simulink model "sampleModel1440"  (R2023a)
settings: Solver=VariableStepAuto  StartTime=0.0  StopTime=10.0  RelTol=1e-3
libraries: hdlsllib x3
settings Model: Creator=user1  LastModifiedBy=user1

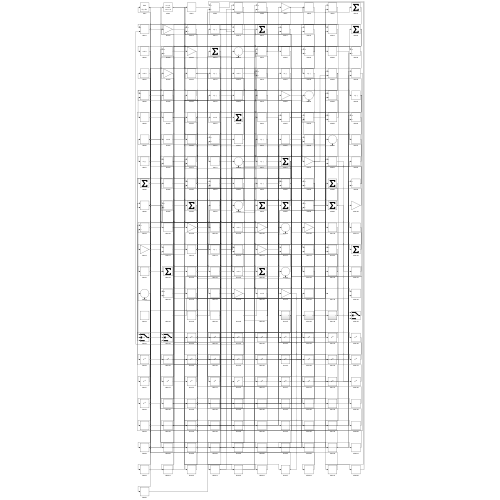
[thumbnail: Simulink's stored preview of the top-level diagram]
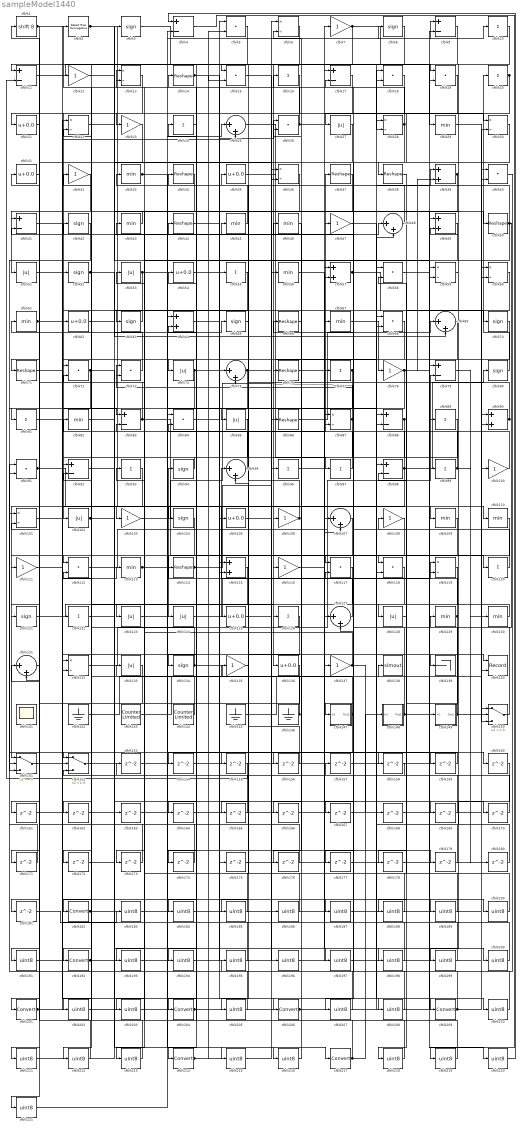
== system sampleModel1440 ==
  cfblk1 : ArithShift  BitShiftNumber=8
  cfblk{10,16,20,24,55,77,81,89,93,96..97,99,120,122,126} (15 alike) : Sum  Inputs=+
  cfblk{7,12,23,32,47,78,100,103,106,108,111,116,135,137} (14 alike) : Gain
  cfblk{6,13,22,28,30,36,59..60,87,101,119,132} (12 alike) : Product  Inputs=*/  RndMeth=Zero  SaturateOnIntegerOverflow=on
  cfblk{27,51,53,74,85,102,123..124,128,133} (10 alike) : Abs  SaturateOnIntegerOverflow=off
  cfblk{3,8,42,52,63,65,70,80,94,104,121,134} (12 alike) : Signum
  cfblk{21,31,35,54,62,105,125,136} (8 alike) : Bias  Bias=0.0  SaturateOnIntegerOverflow=off
  cfblk{25,48,69,75,95,107,127,131} (8 alike) : Sum  Inputs=|++
  cfblk{29,33,43,45..46,56,61,67,82,109..110,113,129..130} (14 alike) : MinMax
  cfblk{4,9,11,17,41,79,83,88,92,98} (10 alike) : Sum  Inputs=+-
  cfblk{5,15,18..19,26,40,58,68,72..73,84,91,112,117..118} (15 alike) : DotProduct  OutDataTypeStr=Inherit: Inherit via internal rule
  cfblk{14,34,37..38,44,50,66,71,76,86,114} (11 alike) : Reshape
  cfblk{39,49,57,64,90,115} (6 alike) : Sum
  cfblk138 : ToWorkspace  VariableName=simout  SaveFormat=Timeseries  SampleTime=-1
  cfblk139 : Terminator
  cfblk140 : Record  FileSettingsInternal="{\"entries\":[{\"content\":{\"excelSettings\":{\"content\":{},\"type\":\"Streamout.ExcelSettings\"}},\"type\":\"Streamout.FileSettingStorage\",\"uuid\":\"\"}],\"packageUris\":[\"http:\\/\\/schema.mathworks.com\\/mf0\\/streamout_blocks\\/R2020a\"],\"version\":\"1.0\"}"  Layout=[1 1]  SignalsInternal="{\"entries\":[{\"content\":{\"signals\":[{\"content\":{\"blockPath\":[],\"dimensions\":[1],\"domain\":\"\",\"lineColor\":\"#a2142f\",\"plots\":[1],\"port\":1,\"signalID\":573,\"signalName\":\"XY Graph:1\"},\"type\":\"RecordBlkView.Signal\",\"uuid\":\"\"},{\"content\":{\"blockPath\":[],\"dimensions\":[1],\"domain\":\"\",\"lineColor\":\"#139fff\",\"plots\":[1],\"port\":2,\"signalID\":576,\"signalName\":\"XY Graph:2\"},\"type\":\"RecordBlkView.Signal\",\"uuid\":\"\"}]},\"type\":\"RecordBlkView.InputSignals\",\"uuid\":\"\"}],\"packageUris\":[\"http:\\/\\/schema.mathworks.com\\/mf0\\/streamout_blocks\\/R2020a\"],\"version\":\"1.0\"}"  VisualizationBindings="{\"xyplotplugin\":{\"info\":[{\"series\":[{\"bindingParametersList\":[{\"parameter\":\"X-Axis\",\"signalID\":573,\"signalName\":\"XY Graph:1\"},{\"parameter\":\"Y-Axis\",\"signalID\":576,\"signalName\":\"XY Graph:2\"}],\"seriesID\":1150}],\"subplotID\":1}]}}"  CompatibilityTag=XY  st=-1
  cfblk141 : Scope
      settings: Floating=on
  cfblk142 : Ground
  cfblk143 : hdlsllib/Sources/Counter Limited  uplimit=7  tsamp=-1
  cfblk144 : hdlsllib/Sources/Counter Limited  uplimit=7  tsamp=-1
  cfblk145 : Ground
  cfblk146 : Ground
  cfblk147 : Subsystem
      settings: LibrarySourceBlock=|
      | hdlsllib/Ports &
      | Subsystems/Subsystem
  cfblk148 : Subsystem
      settings: LibrarySourceBlock=|
      | hdlsllib/Ports &
      | Subsystems/Subsystem
  cfblk149 : Subsystem
      settings: LibrarySourceBlock=|
      | hdlsllib/Ports &
      | Subsystems/Subsystem
  cfblk150 : Switch  SaturateOnIntegerOverflow=off  InputSameDT=off
  cfblk151 : Switch  SaturateOnIntegerOverflow=off  InputSameDT=off
  cfblk152 : Switch  SaturateOnIntegerOverflow=off  InputSameDT=off
  cfblk{153..181} (29 alike) : Delay  SampleTime=1
  cfblk{182,192,201,204,206,209,214,217} (8 alike) : DataTypeConversion  SaturateOnIntegerOverflow=off  RndMeth=Floor
  cfblk{183..191,193..200,202..203,205,207..208,210..213,215..216,218..221} (32 alike) : DataTypeConversion  OutDataTypeStr=uint8  SaturateOnIntegerOverflow=off  RndMeth=Floor
  cfblk2 : hdlsllib/Logic and Bit Operations/Detect Rise Nonnegative  vinit=0  OutDataTypeStr=boolean
  wires:
  cfblk80/1 -> cfblk20/1
  cfblk25/1 -> cfblk97/1
  cfblk108/1 -> cfblk151/1
  cfblk79/1 -> cfblk130/1
  cfblk124/1 -> cfblk119/1
  cfblk104/1 -> cfblk124/1
  cfblk19/1 -> cfblk102/1
  cfblk86/1 -> cfblk69/1
  cfblk106/1 -> cfblk103/1, cfblk35/1
  cfblk85/1 -> cfblk134/1
  cfblk48/1 -> cfblk34/1
  cfblk27/1 -> cfblk136/1
  cfblk99/1 -> cfblk37/1, cfblk180/1
  cfblk39/1 -> cfblk119/2, cfblk74/1
  cfblk134/1 -> cfblk138/1, cfblk22/2
  cfblk59/1 -> cfblk11/1
  cfblk56/1 -> cfblk137/1
  cfblk98/1 -> cfblk80/1, cfblk99/1, cfblk87/1, cfblk221/1
  cfblk8/1 -> cfblk76/1
  cfblk113/1 -> cfblk8/1, cfblk87/2, cfblk159/1
  cfblk2/1 -> cfblk106/1, cfblk36/2
  cfblk67/1 -> cfblk78/1
  cfblk93/1 -> cfblk111/1
  cfblk112/1 -> cfblk7/1
  cfblk83/1 -> cfblk120/1, cfblk61/1
  cfblk50/1 -> cfblk129/1, cfblk26/2, cfblk177/1, cfblk193/1
  cfblk127/1 -> cfblk94/1
  cfblk81/1 -> cfblk83/1
  cfblk143/1 -> cfblk100/1
  cfblk146/1 -> cfblk83/2, cfblk12/1
  cfblk14/1 -> cfblk15/2, cfblk160/1
  cfblk142/1 -> cfblk79/1
  cfblk37/1 -> cfblk123/1
  cfblk88/1 -> cfblk115/2, cfblk173/1
  cfblk103/1 -> cfblk36/1
  cfblk90/1 -> cfblk77/1, cfblk41/2
  cfblk36/1 -> cfblk114/1
  cfblk95/1 -> cfblk53/1
  cfblk82/1 -> cfblk217/1
  cfblk129/1 -> cfblk95/1, cfblk108/1, cfblk158/1
  cfblk117/1 -> cfblk152/1
  cfblk11/1 -> cfblk19/1
  cfblk132/1 -> cfblk79/2
  cfblk35/1 -> cfblk88/1
  cfblk16/1 -> cfblk23/1
  cfblk102/1 -> cfblk109/1, cfblk44/1
  cfblk42/1 -> cfblk151/3
  cfblk152/1 -> cfblk59/1
  cfblk78/1 -> cfblk10/1, cfblk39/2, cfblk166/1
  cfblk10/1 -> cfblk28/2
  cfblk30/1 -> cfblk121/1
  cfblk75/1 -> cfblk48/1, cfblk194/1
  cfblk53/1 -> cfblk63/1, cfblk25/1
  cfblk32/1 -> cfblk51/1
  cfblk63/1 -> cfblk62/1
  cfblk49/1 -> cfblk117/1
  cfblk6/1 -> cfblk214/1
  cfblk24/1 -> cfblk204/1
  cfblk107/1 -> cfblk192/1
  cfblk45/1 -> cfblk33/1
  cfblk66/1 -> cfblk116/1
  cfblk43/1 -> cfblk41/1
  cfblk65/1 -> cfblk45/1
  cfblk34/1 -> cfblk81/1
  cfblk148/1(Out1) -> cfblk13/1, cfblk220/1
  cfblk97/1 -> cfblk32/1
  cfblk151/1 -> cfblk113/1
  cfblk26/1 -> cfblk2/1, cfblk30/1
  cfblk29/1 -> cfblk150/3
  cfblk1/1 -> cfblk21/1, cfblk139/1
  cfblk9/1 -> cfblk71/1
  cfblk20/1 -> cfblk85/1, cfblk38/1
  cfblk22/1 -> cfblk50/1
  cfblk60/1 -> cfblk118/1
  cfblk137/1 -> cfblk43/1, cfblk168/1
  cfblk105/1 -> cfblk140/1
  cfblk87/1 -> cfblk75/2, cfblk176/1
  cfblk61/1 -> cfblk104/1, cfblk25/2
  cfblk91/1 -> cfblk125/1, cfblk110/1
  cfblk18/1 -> cfblk201/1
  cfblk74/1 -> cfblk26/1, cfblk203/1
  cfblk130/1 -> cfblk128/1
  cfblk3/1 -> cfblk15/1
  cfblk73/1 -> cfblk31/1
  cfblk62/1 -> cfblk46/1
  cfblk145/1 -> cfblk19/2
  cfblk5/1 -> cfblk52/1
  cfblk33/1 -> cfblk88/2, cfblk216/1
  cfblk28/1 -> cfblk16/1, cfblk27/1, cfblk147/1(In1)
  cfblk57/1 -> cfblk149/1(In1), cfblk39/1
  cfblk114/1 -> cfblk56/1, cfblk89/1
  cfblk147/1(Out1) -> cfblk13/2, cfblk164/1, cfblk165/1
  cfblk120/1 -> cfblk66/1
  cfblk121/1 -> cfblk126/1
  cfblk72/1 -> cfblk91/2, cfblk197/1
  cfblk94/1 -> cfblk92/1
  cfblk44/1 -> cfblk105/1
  cfblk101/1 -> cfblk206/1
  cfblk118/1 -> cfblk127/2
  cfblk68/1 -> cfblk182/1
  cfblk149/1(Out1) -> cfblk90/1, cfblk42/1
  cfblk150/1 -> cfblk98/2
  cfblk7/1 -> cfblk29/1, cfblk155/1
  cfblk77/1 -> cfblk112/1, cfblk73/2, cfblk154/1
  cfblk111/1 -> cfblk152/2
  cfblk12/1 -> cfblk59/2
  cfblk100/1 -> cfblk73/1
  cfblk144/1 -> cfblk93/1
  cfblk58/1 -> cfblk49/1
  cfblk92/1 -> cfblk65/1
  cfblk69/1 -> cfblk132/2
  cfblk41/1 -> cfblk72/1
  cfblk52/1 -> cfblk70/1, cfblk69/2
  cfblk116/1 -> cfblk67/1
  cfblk54/1 -> cfblk9/1
  cfblk47/1 -> cfblk209/1
  cfblk153/1 -> cfblk127/1
  cfblk155/1 -> cfblk11/2
  cfblk46/1 -> cfblk156/1
  cfblk156/1 -> cfblk95/2
  cfblk157/1 -> cfblk58/1
  cfblk158/1 -> cfblk152/3
  cfblk159/1 -> cfblk151/2
  cfblk23/1 -> cfblk161/1
  cfblk161/1 -> cfblk75/1
  cfblk136/1 -> cfblk162/1
  cfblk162/1 -> cfblk28/1
  cfblk163/1 -> cfblk5/1
  cfblk164/1 -> cfblk48/2
  cfblk165/1 -> cfblk92/2
  cfblk166/1 -> cfblk90/2
  cfblk119/1 -> cfblk167/1
  cfblk167/1 -> cfblk118/2
  cfblk168/1 -> cfblk60/1
  cfblk125/1 -> cfblk169/1
  cfblk169/1 -> cfblk57/1
  cfblk122/1 -> cfblk170/1
  cfblk170/1 -> cfblk17/1
  cfblk133/1 -> cfblk171/1
  cfblk171/1 -> cfblk91/1
  cfblk89/1 -> cfblk172/1
  cfblk173/1 -> cfblk1/1
  cfblk115/1 -> cfblk174/1
  cfblk174/1 -> cfblk22/1
  cfblk175/1 -> cfblk150/2
  cfblk176/1 -> cfblk112/2
  cfblk177/1 -> cfblk117/2
  cfblk38/1 -> cfblk178/1
  cfblk178/1 -> cfblk150/1
  cfblk123/1 -> cfblk179/1
  cfblk179/1 -> cfblk98/1
  cfblk180/1 -> cfblk49/2
  cfblk31/1 -> cfblk181/1
  cfblk182/1 -> cfblk57/2, cfblk140/2
  cfblk181/1 -> cfblk183/1
  cfblk183/1 -> cfblk68/1
  cfblk70/1 -> cfblk184/1
  cfblk184/1 -> cfblk68/2
  cfblk135/1 -> cfblk185/1
  cfblk185/1 -> cfblk153/1
  cfblk186/1 -> cfblk135/1
  cfblk64/1 -> cfblk187/1
  cfblk187/1 -> cfblk157/1
  cfblk128/1 -> cfblk188/1
  cfblk188/1 -> cfblk64/1
  cfblk51/1 -> cfblk189/1
  cfblk189/1 -> cfblk64/2
  cfblk96/1 -> cfblk190/1
  cfblk190/1 -> cfblk58/2
  cfblk21/1 -> cfblk191/1
  cfblk191/1 -> cfblk96/1
  cfblk192/1 -> cfblk175/1, cfblk115/1, cfblk72/2
  cfblk193/1 -> cfblk107/1
  cfblk194/1 -> cfblk107/2
  cfblk40/1 -> cfblk195/1
  cfblk195/1 -> cfblk132/1
  cfblk15/1 -> cfblk196/1
  cfblk196/1 -> cfblk40/1
  cfblk197/1 -> cfblk40/2
  cfblk84/1 -> cfblk198/1
  cfblk198/1 -> cfblk14/1
  cfblk160/1 -> cfblk199/1
  cfblk199/1 -> cfblk84/1
  cfblk76/1 -> cfblk200/1
  cfblk200/1 -> cfblk84/2
  cfblk201/1 -> cfblk122/1, cfblk3/1
  cfblk17/1 -> cfblk202/1
  cfblk202/1 -> cfblk18/1
  cfblk203/1 -> cfblk18/2
  cfblk204/1 -> cfblk86/1, cfblk55/1
  cfblk126/1 -> cfblk205/1
  cfblk205/1 -> cfblk24/1
  cfblk206/1 -> cfblk9/2, cfblk60/2
  cfblk109/1 -> cfblk207/1
  cfblk207/1 -> cfblk101/1
  cfblk154/1 -> cfblk208/1
  cfblk208/1 -> cfblk101/2
  cfblk209/1 -> cfblk30/2, cfblk17/2
  cfblk71/1 -> cfblk210/1
  cfblk210/1 -> cfblk47/1
  cfblk131/1 -> cfblk211/1
  cfblk211/1 -> cfblk163/1
  cfblk13/1 -> cfblk212/1
  cfblk212/1 -> cfblk131/1
  cfblk55/1 -> cfblk213/1
  cfblk213/1 -> cfblk131/2
  cfblk214/1 -> cfblk186/1, cfblk5/2
  cfblk172/1 -> cfblk215/1
  cfblk215/1 -> cfblk6/1
  cfblk216/1 -> cfblk6/2
  cfblk217/1 -> cfblk133/1, cfblk148/1(In1)
  cfblk110/1 -> cfblk218/1
  cfblk218/1 -> cfblk82/1
  cfblk4/1 -> cfblk219/1
  cfblk219/1 -> cfblk54/1
  cfblk220/1 -> cfblk4/1
  cfblk221/1 -> cfblk4/2

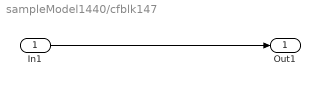
== system sampleModel1440/cfblk147 ==
  In1 : Inport
  Out1 : Outport
  wires:
  In1/1 -> Out1/1

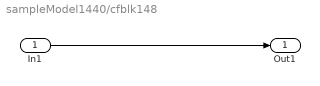
== system sampleModel1440/cfblk148 ==
  In1 : Inport
  Out1 : Outport
  wires:
  In1/1 -> Out1/1

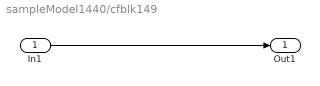
== system sampleModel1440/cfblk149 ==
  In1 : Inport
  Out1 : Outport
  wires:
  In1/1 -> Out1/1
